simulink model "SnakeSymul"  (R2024b)
settings: Solver=VariableStepAuto  StartTime=0.0  StopTime=10.0  RelTol=1e-3
InitFcn:
  | N  = 14;                                      % Number of snake robot links
  | m  = 0.406;                                   % Weight of snake robot link
  | l  = 0.0525;                                  % Radius of snake robot link
  | g  = 9.81;                                    % Gravitational acceleration
  | diameter = 0.30;                              % Diameter of a pipeline
  | diameterInfluence = 0.10;                     % Auxiliary constant
  | pipeLength = 3;                                     % Length of a pipeline
  | d = param.diameter - 2*l;               % Theoretical diameter for snake robot links
  | shotsNumber = 50;                                   % Auxiliary variable for animation
  | dt = 0.01;                                    % Time increment [s]
  | 
  | ct = 0.015;                                   % Viscous friction coefphicient of a ground in tangental direction
  | cn = 0.03;                                    % Viscous friction coefphicient of a ground in normal direction
  | ut = 0.15;                                    % Coulomb friction coefphicient of a ground in tangental direction
  | un = 0.3;                                     % Coulomb friction coefphicient of a ground in normal direction
  | ctPipe = 0.08;                                % Viscous friction coefphicient of a pipeline in tangental direction
  | utPipe = 0.2;                                 % Coulomb friction coefphicient of a pipeline in tangental direction
  | umax = 3;                                     % Maximum snake robot link torque
  | qmax = 400*param.dt;                          % Contact parameter
  | Erub = 400000;                                % Contact parameter
  | vrub = 0.49;                                  % Contact parameter
  | friction = 1;                                 % Choice of friction:   0 - Coulomb, 1 - viscous
  | contact = 0;                                  % Choice of side walls contact: 0 - without contact, 1 - with contact
  | minLinkVel = 0.001;                           % Auxiliary variable of snake robot link angular velocity
  | Plot3D = 0;                                   % Choice of a graph:    0 - 2D, 1 - 3D
  | resultsShow = 1;                              % Choice of animation:  0 - show simulation, 1 - show graphs
  | % Controler parameters:
  | kp  = 25;                                     % Gain for position controller
  | kd  = 10;                                     % Gain for velocity controller
  | % Simulation time:
  | t=0:param.dt:30;
  | 
  | % Reference trajectory parameters:
  | alpha = 0.3981;
  | omega = 0.6936;
  | delta = 0.4914;
  | offset = 0;
settings Model: Creator=maniente  LastModifiedBy=maniente

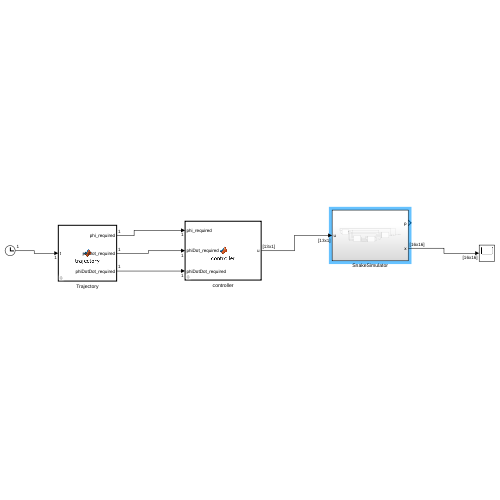
[thumbnail: Simulink's stored preview of the top-level diagram]
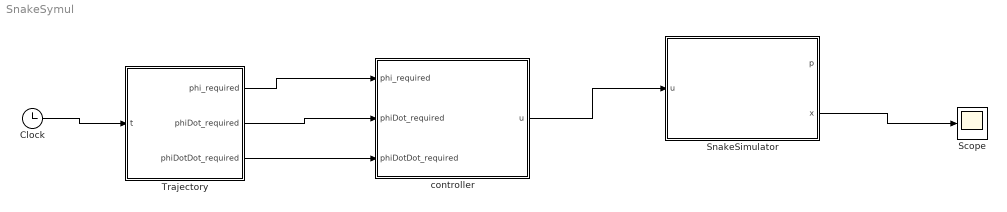
== system SnakeSymul ==
  Clock : Clock
  Scope : Scope
  SnakeSimulator : Subsystem
  Trajectory : MATLAB Function  TreatAsAtomicUnit=on  mask{alpha=alpha, omega=omega, delta=delta, offset=offset, N=N}
      mask prompts: N "number of links"
  controller : MATLAB Function  TreatAsAtomicUnit=on  mask{N=N, kp=kp, kd=kd, umax=umax}
      mask prompts: N "number of links"; umax "Saturation value"
  wires:
  Trajectory/1(phi_required) -> controller/1(phi_required)
  Trajectory/2(phiDot_required) -> controller/2(phiDot_required)
  Trajectory/3(phiDotDot_required) -> controller/3(phiDotDot_required)
  controller/1(u) -> SnakeSimulator/1(u)
  SnakeSimulator/2(x) -> Scope/1
  Clock/1 -> Trajectory/1(t)

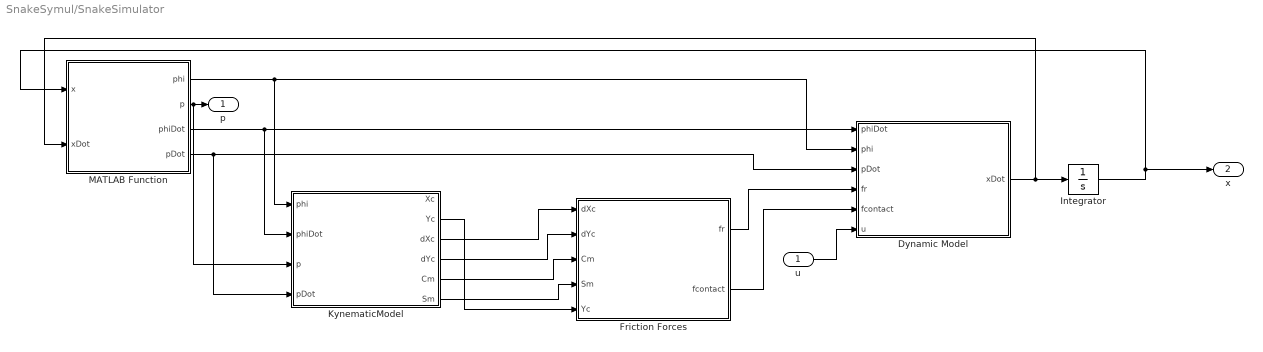
== system SnakeSymul/SnakeSimulator ==
  u : Inport
  Dynamic Model : MATLAB Function  TreatAsAtomicUnit=on  mask{N=N, l=l, m=m}
      mask prompts: N "number of Links"; l "lenght of 1 link"; m "mass of 1 link"
  Friction Forces : MATLAB Function  TreatAsAtomicUnit=on  mask{viscous=friction, ut=ut, un=un, ct=ct, cn=cn, m=m, l=l, d=diameter, ctPipe=ctPipe, utPipe=utPipe, minLinkVel=minLinkVel, contact=contact, Erub=Erub, vrub=vrub, N=N}
      mask prompts: viscous "viscouse friction flag(1 viscous , 0 coulomb)"; ut "Coulomb friction coefphicient of a ground in tangential direction"; un "Coulomb friction coefphicient of a ground in normal direction"; ct "Viscous friction coefphicient of a ground in tangental direction"; cn "Viscous friction coefphicient of a ground in normal direction"; m "Weight of snake robot link"; l "link lenght"; d "diameter"; ctPipe "ct pipe"; utPipe "ut pipe"; contact "contact flag for a x-axis pipe"; N "number of links"
  Integrator : Integrator  InitialCondition=zeros(N+2)
  KynematicModel : MATLAB Function  TreatAsAtomicUnit=on  mask{N=N, l=l}
      mask prompts: N "Number of snake robot links"; l "Radius of snake robot link length"
  MATLAB Function : MATLAB Function  TreatAsAtomicUnit=on  mask{N=N}
      mask prompts: N "number of links"
  p : Outport
  x : Outport  Port=2
  wires:
  u/1 -> Dynamic Model/6(u)
  Integrator/1 -> x/1, MATLAB Function/1(x)
  Dynamic Model/1(xDot) -> MATLAB Function/2(xDot), Integrator/1
  KynematicModel/6(Sm) -> Friction Forces/4(Sm)
  MATLAB Function/2(p) -> KynematicModel/3(p), p/1
  KynematicModel/2(Yc) -> Friction Forces/5(Yc)
  MATLAB Function/4(pDot) -> KynematicModel/4(pDot), Dynamic Model/3(pDot)
  MATLAB Function/3(phiDot) -> KynematicModel/2(phiDot), Dynamic Model/1(phiDot)
  KynematicModel/5(Cm) -> Friction Forces/3(Cm)
  KynematicModel/3(dXc) -> Friction Forces/1(dXc)
  KynematicModel/4(dYc) -> Friction Forces/2(dYc)
  Friction Forces/1(fr) -> Dynamic Model/4(fr)
  Friction Forces/2(fcontact) -> Dynamic Model/5(fcontact)
  MATLAB Function/1(phi) -> KynematicModel/1(phi), Dynamic Model/2(phi)

== matlab function SnakeSymul/Trajectory ==
  data: phi_required output; phiDot_required output; phiDotDot_required output; offset parameter; delta parameter; omega parameter; alpha parameter; N parameter; t input
function [phi_required,phiDot_required,phiDotDot_required] = trajectory(offset, delta, omega, alpha,N,t)

for i=1:N-1
    phi_required         = alpha*sin((omega*t+(i-1)*delta)) + offset;
        phiDot_required      = alpha*omega*cos((omega*t+(i-1)*delta));
        phiDotDot_required   = -alpha*omega*omega*sin((omega*t+(i-1)*delta));
end

== matlab function SnakeSymul/controller ==
  data: phi_required input; phiDot_required input; phiDotDot_required input; u output size=[N-1 1]; N parameter; kp parameter; kd parameter; umax parameter
function u  = controller(phi_required,phiDot_required,phiDotDot_required,N, kp, kd, umax)
    u = zeros(N-1,1);
    for i=1:N-1
            u(i,1)              = phiDotDot_required + kp*(phi_required - phi(i)) + kd*(phiDot_required - phiDot(i));
            if(u(i,1)>umax)
                u(i,1) = umax;
            elseif(u(i,1)<-umax)
                u(i,1) = -umax;
            end
    end

== matlab function SnakeSymul/SnakeSimulator/Friction Forces ==
  data: dXc input; dYc input; Cm input; Sm input; fr output; viscous parameter; g parameter; ut parameter; un parameter; ct parameter; cn parameter; m parameter; minLinkVel parameter; vrub parameter size=1; Erub parameter size=1; l parameter; d parameter; ctPipe parameter; utPipe parameter; contact parameter; fcontact output size=[2*N, 1]; Yc input size=[N 1]; N parameter
function [fr,fcontact]  = frictionForces(dXc, dYc, Cm, Sm, viscous, g, ut, un, ct, cn, m, ...
                                        minLinkVel, vrub, Erub, l, d, ctPipe, utPipe, contact, Yc,N)
%% Friction
    % ==============================================================================================================
    % Viscous
    if(viscous==1)
        fr = -[ct*(Cm*Cm)+cn*(Sm*Sm), (ct-cn)*Sm*Cm;(ct-cn)*Sm*Cm, ct*(Sm*Sm)+cn*(Cm*Cm)]*[dXc;dYc];
    else     
    % Coulomb
        fr = -m*g*[ut*Cm, -un*Sm;ut*Sm, un*Cm]*sign([Cm, Sm;-Sm, Cm]*[dXc;dYc]);
    end
 
% ==============================================================================================================
    %% Contact model
    % ==============================================================================================================
    fct = zeros(N,1);
    fcn = zeros(N,1);
    fctBo1l = zeros(N,1);

    if contact == 1
        for i1=1:N
            fcn(i1,1) = 0;
            fctBo1l(i1,1) = 0;
            fct(i1,1) = 0;
        end
        
        for i1=1:N  

            if((Yc(i1)>=(d/2)))
                fcn(i1,1) = -(sqrt((16*Erub*2*l)/(9*(1-vrub^2))))*((abs(Yc(i1))-(d/2))^(3/2));
                if(abs(dXc(i1))>minLinkVel)
                    fctBo1l(i1,1) = 1;
                    if(viscous == 1) 
                        fct(i1,1) = fctBo1l(i1)*ctPipe*sign(-dXc(i1));
                    else
                        fct(i1,1) = fctBo1l(i1)*(abs(fcn(i1))*utPipe*sign(-dXc(i1)));
                    end
                else
                    fctBo1l(i1,1) = 0;
                    fct(i1,1) = 0;
                end
            elseif((Yc(i1)<=(-d/2)))
                fcn(i1,1) = (sqrt((16*Erub*2*l)/(9*(1-vrub^2))))*((abs(Yc(i1))-(d/2))^(3/2));
                if(abs(dXc(i1))>minLinkVel)
                    fctBo1l(i1,1) = 1;
                    if(viscous == 1)
                        fct(i1,1) = fctBo1l(i1)*ctPipe*sign(-dXc(i1));
                    else
                        fct(i1,1) = fctBo1l(i1)*(abs(fcn(i1))*utPipe*sign(-dXc(i1)));
                    end
                else
                    fctBo1l(i1,1) = 0;
                    fct(i1,1) = 0;
                end
            else
                fcn(i1,1) = 0;
                fctBo1l(i1,1) = 0;
                fct(i1,1) = 0;
            end
            
        end

    end

fcontact = [fct; fcn];  % <== assign this unconditionally at the end
end

== matlab function SnakeSymul/SnakeSimulator/KynematicModel ==
  data: phi input; phiDot input; p input; pDot input; Xc output size=[N 1]; Yc output size=[N 1]; dXc output size=[N 1]; dYc output size=[N 1]; Cm output size=[N N]; Sm output size=[N N]; N parameter; l parameter
function [Xc, Yc, dXc, dYc, Cm, Sm] = kinematicModel(phi,phiDot,p,pDot,N, l)

%#codegen
Xc   = zeros(N,1);
Yc   = zeros(N,1);
dXc  = zeros(N,1);
dYc  = zeros(N,1);
Cm   = zeros(N,N);
Sm   = zeros(N,N);

% ==============================================================================================================
%% Basic parameters
% ==============================================================================================================
A       = eye(N-1,N) + diag(ones(N-2,1),1);         % A: N-1 × N with 1s on the diagonal and superdiagonal
D       = eye(N-1,N) - diag(ones(N-2,1),1);         % D: N-1 × N with 1s on diag, -1s on superdiag
J       = -eye(N,N+1) + diag(ones(N,1),1);          % J: N × (N+1), -1 on diag, 1 on superdiag
K       = eye(N,N+1);                               % K: N × (N+1), ones on diag
J2      = eye(N,N-1) + diag(ones(N-1,1),-1);        % J2: N × (N-1), 1 on diag and subdiag
Jf      = eye(N,N-1) - diag(ones(N-1,1),-1);        % Jf: N × (N-1), 1 on diag, -1 on subdiag

HH      = triu(ones(N));                            % Upper triangular matrix of ones
e       = [ones(N,1); 0];                           % Vector of ones with last element 0 (N+1 × 1)
k       = ones(N,1);                                
j       = zeros(N,1); j(end) = -1;                  % j: N × 1 with -1 at last position

Cm      = diag(zeros(N,1));
Sm      = diag(zeros(N,1));
% ==============================================================================================================
%% Kinematic model
% ==============================================================================================================
theta       = HH * phi;
thetaDot    = HH * phiDot;

s_vect      = sin(theta);
c_vect      = cos(theta);

Cm = diag(c_vect);
Sm = diag(s_vect);

A = J*J';
B = (1/N)*j;
C = (1/N)*j';
D = (1/N);

DD = inv(D - C / A * B);
AA = inv(A) + A / B * DD * C / A;
BB = -A / B * DD;
CC = -DD * C / A;

Hinv = [J' (1/N)*e] * [AA BB; CC DD];

X = Hinv * [2*l*c_vect; p(1) - (l/N)*k'*c_vect];
Y = Hinv * [2*l*s_vect; p(2) - (l/N)*k'*s_vect];

dX = -J'*AA*2*l*Sm*thetaDot - (1/N)*e*CC*2*l*Sm*thetaDot + ...
      J'*BB*pDot(1) + J'*BB*(l/N)*k'*Sm*thetaDot + ...
      (1/N)*e*DD*pDot(1) + (1/N)*e*DD*(l/N)*k'*Sm*thetaDot;

dY =  J'*AA*2*l*Cm*thetaDot + (1/N)*e*CC*2*l*Cm*thetaDot + ...
      J'*BB*pDot(2) - J'*BB*(l/N)*k'*Cm*thetaDot + ...
      (1/N)*e*DD*pDot(2) - (1/N)*e*DD*(l/N)*k'*Cm*thetaDot;

Xc = K * X + l * c_vect;
Yc = K * Y + l * s_vect;

dXc = K * dX - l * Sm * thetaDot;
dYc = K * dY + l * Cm * thetaDot;

== matlab function SnakeSymul/SnakeSimulator/Dynamic Model ==
  data: phiDot input; phi input; pDot input; fr input; fcontact input; u input size=[N-1 1]; xDot output; N parameter; l parameter; m parameter
function xDot = snakeDynamics(phiDot,phi, pDot,fr,fcontact,u,N, l, m)
    I = (m*(2*l)^2)/3;                          % Moment of inertia
   % ==============================================================================================================
    %% Auxiliary matrices
    % ==============================================================================================================
    A = diag(ones(N-1,1), 0) + diag(ones(N-2,1), 1);
    D = diag(ones(N-1,1), 0) - diag(ones(N-2,1), 1);
    
    Va= A'/(D*D')*A;
    Ka = A'/(D*D')*D;
    HH = ones(N,N);
    HH = triu(HH);

    theta = HH*phi;
    
    Cm = diag(cos(theta));
    Sm = diag(sin(theta));

    
    
    k = ones(1,N)';   
    % ================================================================================================
    %% Dynamic model
    % ==============================================================================================================

    M = I*eye(N) + m*l*l*Sm*Va*Sm + m*l*l*Cm*Va*Cm;
    W = m*l*l*Sm*Va*Cm - m*l*l*Cm*Va*Sm;

    i1M = [HH'*M*HH zeros(N,2);zeros(2,N) N*m*eye(2,2)];
    WWW = [HH'*W*diag(HH*phiDot)*HH*phiDot;zeros(2,1)];
    GGG = [-l*HH'*Sm*Ka l*HH'*Cm*Ka;-k' zeros(1,N);zeros(1,N) -k'];
    BBB = [eye(N-1,N-1);zeros(3,N-1)];

    i11 = i1M(1:N-1,1:N-1);
    i12 = i1M(1:N-1,N:N+2);
    M21 = i1M(N:N+2,1:N-1);
    M22 = i1M(N:N+2,N:N+2);
    W1  = WWW(1:N-1);
    W2  = WWW(N:N+2);
    G1  = GGG(1:N-1,1:2*N);
    G2  = GGG(N:N+2,1:2*N);

    Aq  = -inv(M22)*(W2 + G2*fr + G2*fcontact);
    Bq  = -inv(M22)*M21;    
    xDot = [phiDot;pDot;u;Aq+Bq*u];

== matlab function SnakeSymul/SnakeSimulator/MATLAB Function ==
  data: x input; xDot input; phi output; p output; phiDot output; pDot output; N parameter
function [phi,p,phiDot,pDot] = stateSplitter(x,xDot,N)
 phi     = x(1:N);
 p       = x(N+1:N+2);
 phiDot  = xDot(1:N);
 pDot    = xDot(N+1:N+2);
